simulink subsystem "TiltEstimation"  (R2024b)
settings: Solver=VariableStepAuto  StartTime=0.0  StopTime=10.0  RelTol=1e-3
values from neighbouring files (symbols this model uses):
  LPFDen = LPF.Denominator{1}    [Plant_balrob_calculations.m]
  LPFNum = LPF.Numerator{1}    [Plant_balrob_calculations.m]
undefined symbols (not defined in the file or in its folder): DiscIntNeverNeededParam
settings Model: Creator=federico  LastModifiedBy=federico

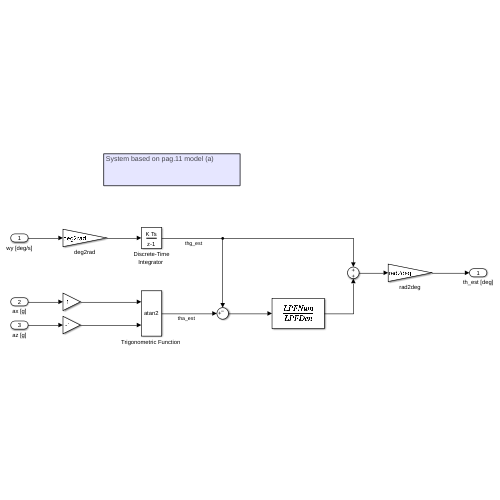
[thumbnail: Simulink's stored preview of the top-level diagram]
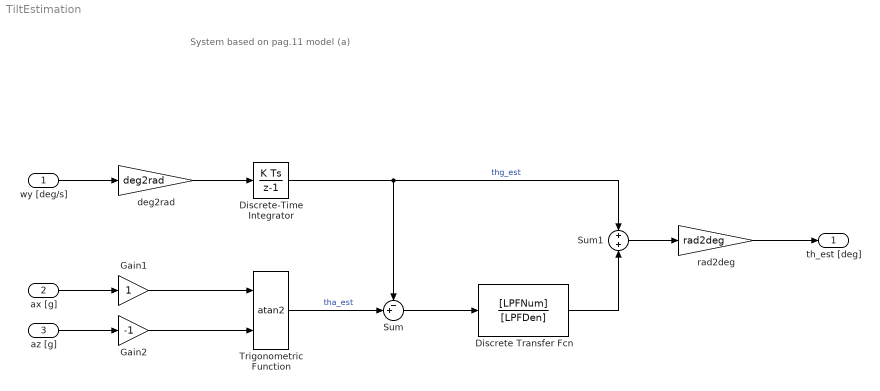
== system TiltEstimation ==
  note: System based on pag.11 model (a)
  wy [deg/s] : Inport
  ax [g] : Inport  Port=2
  az [g] : Inport  Port=3
  Discrete Transfer Fcn : DiscreteTransferFcn  Numerator=[LPFNum]  Denominator=[LPFDen]
  "Discrete-Time Integrator " : DiscreteIntegrator  SampleTime=-1  ICPrevOutput=DiscIntNeverNeededParam  ICPrevScaledInput=DiscIntNeverNeededParam
  Gain1 : Gain
  Gain2 : Gain  Gain=-1
  Sum : Sum  Inputs=-+|
  Sum1 : Sum  Inputs=+|+
  "Trigonometric Function " : Trigonometry  Operator=atan2
  deg2rad : Gain  Gain=deg2rad
  rad2deg : Gain  Gain=rad2deg
  th_est [deg] : Outport
  wires:
  wy [deg/s]/1 -> deg2rad/1
  ax [g]/1 -> Gain1/1
  az [g]/1 -> Gain2/1
  deg2rad/1 -> "Discrete-Time Integrator "/1
  Gain1/1 -> "Trigonometric Function "/1
  Gain2/1 -> "Trigonometric Function "/2
  "Trigonometric Function "/1 -> Sum/2  "tha_est"
  Sum/1 -> Discrete Transfer Fcn/1
  Sum1/1 -> rad2deg/1
  rad2deg/1 -> th_est [deg]/1
  Discrete Transfer Fcn/1 -> Sum1/2
  "Discrete-Time Integrator "/1 -> Sum/1, Sum1/1  "thg_est"
